simulink model "q_6"  (R2020a)
settings: Solver=VariableStepAuto  StartTime=0.0  StopTime=10.0  RelTol=1e-3
settings Model: Creator=Admin  LastModifiedBy=Admin

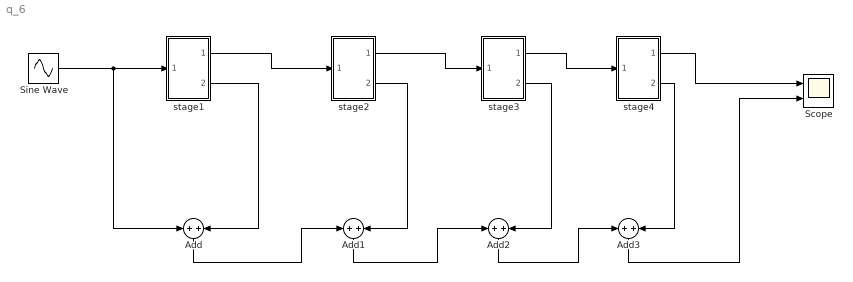
== system q_6 ==
  Add{,1..3} (4 alike) : Sum
  Scope : Scope  NumInputPorts=2
  Sine Wave : Sin  Frequency=2*pi  SampleTime=0
  stage1 : Subsystem
  stage2 : Subsystem
  stage3 : Subsystem
  stage4 : Subsystem
  wires:
  Sine Wave/1 -> Add/1, stage1/1(In1)
  Add/1 -> Add1/1
  Add1/1 -> Add2/1
  Add2/1 -> Add3/1
  Add3/1 -> Scope/2
  stage1/2(Out2) -> Add/2
  stage1/1(Out1) -> stage2/1(In1)
  stage2/2(Out2) -> Add1/2
  stage2/1(Out1) -> stage3/1(In1)
  stage3/2(Out2) -> Add2/2
  stage3/1(Out1) -> stage4/1(In1)
  stage4/1(Out1) -> Scope/1
  stage4/2(Out2) -> Add3/2

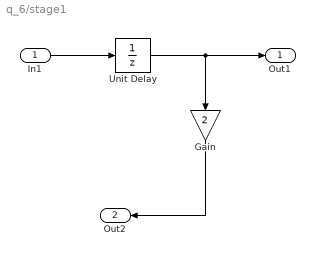
== system q_6/stage1 ==
  In1 : Inport
  Gain : Gain  Gain=2
  Unit Delay : UnitDelay  SampleTime=-1  HasFrameUpgradeWarning=on
  Out1 : Outport
  Out2 : Outport  Port=2
  wires:
  Unit Delay/1 -> Out1/1, Gain/1
  In1/1 -> Unit Delay/1
  Gain/1 -> Out2/1

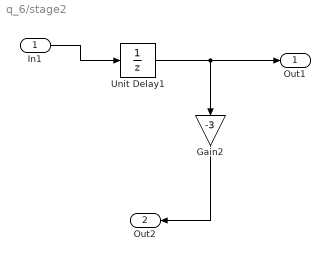
== system q_6/stage2 ==
  In1 : Inport
  Gain2 : Gain  Gain=-3
  Unit Delay1 : UnitDelay  SampleTime=-1  HasFrameUpgradeWarning=on
  Out1 : Outport
  Out2 : Outport  Port=2
  wires:
  In1/1 -> Unit Delay1/1
  Unit Delay1/1 -> Out1/1, Gain2/1
  Gain2/1 -> Out2/1

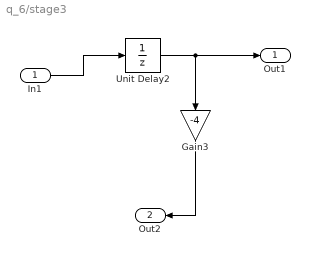
== system q_6/stage3 ==
  In1 : Inport
  Gain3 : Gain  Gain=-4
  Unit Delay2 : UnitDelay  SampleTime=-1  HasFrameUpgradeWarning=on
  Out1 : Outport
  Out2 : Outport  Port=2
  wires:
  Unit Delay2/1 -> Out1/1, Gain3/1
  In1/1 -> Unit Delay2/1
  Gain3/1 -> Out2/1

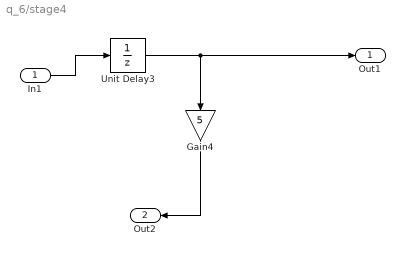
== system q_6/stage4 ==
  In1 : Inport
  Gain4 : Gain  Gain=5
  Unit Delay3 : UnitDelay  SampleTime=-1  HasFrameUpgradeWarning=on
  Out1 : Outport
  Out2 : Outport  Port=2
  wires:
  Unit Delay3/1 -> Out1/1, Gain4/1
  In1/1 -> Unit Delay3/1
  Gain4/1 -> Out2/1
